simulink model "Maltab2Simulink"  (R2017a)
settings: Solver=VariableStepAuto  StartTime=0.0  StopTime=10.0  RelTol=1e-3
settings Model: Creator=Huang Guoming  LastModifiedBy=Huang Guoming

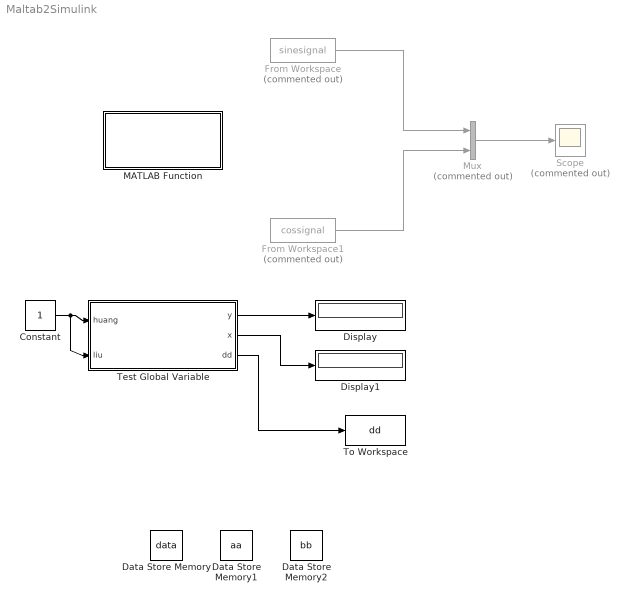
== system Maltab2Simulink ==
  Constant : Constant
  Data Store Memory : DataStoreMemory  DataStoreName=data  ReadBeforeWriteMsg=warning  WriteAfterWriteMsg=warning  WriteAfterReadMsg=warning  ShowAdditionalParam=off  OutDataTypeStr=double
  Data Store Memory1 : DataStoreMemory  DataStoreName=aa  ReadBeforeWriteMsg=warning  WriteAfterWriteMsg=warning  WriteAfterReadMsg=warning  ShowAdditionalParam=off  OutDataTypeStr=double
  Data Store Memory2 : DataStoreMemory  DataStoreName=bb  ReadBeforeWriteMsg=warning  WriteAfterWriteMsg=warning  WriteAfterReadMsg=warning  InitialValue=[0;0;0]  ShowAdditionalParam=off  OutDataTypeStr=double
  Display : Display
  Display1 : Display
  From Workspace : FromWorkspace  Commented=on  VariableName=sinesignal  SampleTime=0
  From Workspace1 : FromWorkspace  Commented=on  VariableName=cossignal  SampleTime=0
  MATLAB Function : MATLAB Function  TreatAsAtomicUnit=on
  Mux : Mux  Commented=on  Inputs=2
  Scope : Scope  Commented=on
  Test Global Variable : MATLAB Function  TreatAsAtomicUnit=on
  To Workspace : ToWorkspace  VariableName=dd  SampleTime=-1
  wires:
  Mux/1 -> Scope/1
  From Workspace/1 -> Mux/1
  From Workspace1/1 -> Mux/2
  Test Global Variable/1(y) -> Display/1
  Test Global Variable/2(x) -> Display1/1
  Constant/1 -> Test Global Variable/2(liu), Test Global Variable/1(huang)
  Test Global Variable/3(dd) -> To Workspace/1

== matlab function Maltab2Simulink/Test Global Variable ==
  data: y output; x output; data data_store_memory; aa data_store_memory; bb data_store_memory; huang input; liu input; dd output
function [y,x,dd] =get_global_varible(huang,liu)

global data aa bb

y = data+10;

data = data + 3;

x = data*5;


tt = (huang +  liu) * bb;

dd = tt';

end

== matlab function Maltab2Simulink/MATLAB Function ==
  data: data data_store_memory; aa data_store_memory; bb data_store_memory
function Parameter_initial

global data aa bb

data = 10;

aa = 2018;

bb = [1; 2; 3];

end
